simulink model "sim_DOF"  (R2020a)
settings: Solver=ode4  StartTime=0  StopTime=t_end  FixedStep=Step_Time  RelTol=1e-3
values from neighbouring files (symbols this model uses):
  A = [ 0 1 ... (first row only)    [hils2.m]    (also in miniHILS_data.m = [ 0 0 1 0; model_DOF.m = 0.003)
  c1 = 140    [model_DOF.m]    (also in model_nonfeedback.m = 7)
  c2 = 1000    [hils2.m]    (also in miniHILS_data.m = 7; model_DOF.m = 37; model_nonfeedback.m = 13)
  Hz = 2*2*pi    (= 12.5663706144)    [model_DOF.m]
  k1 = 180000    [hils2.m]    (also in miniHILS_data.m = 2200; model_DOF.m = 2200; model_nonfeedback.m = 2200)
  k2 = 30000    [hils2.m]    (also in miniHILS_data.m = 405; model_DOF.m = 405; model_nonfeedback.m = 405)
  m1 = 30.0    (= 30)    [hils2.m]    (also in miniHILS_data.m = 1.5; model_DOF.m = 1.5; model_nonfeedback.m = 1.5)
  m2 = 300.0    (= 300)    [hils2.m]    (also in miniHILS_data.m = 6.4; model_DOF.m = 6.4; model_nonfeedback.m = 6.4)
  T_diff = 1/(2*pi*cutoff)    (= 0.00795774715459)    [miniHILS_data.m]    (also in model_DOF.m = 0.00198943678865)
settings Model: Creator=Peanatsu  LastModifiedBy=Natsu Nakagawa

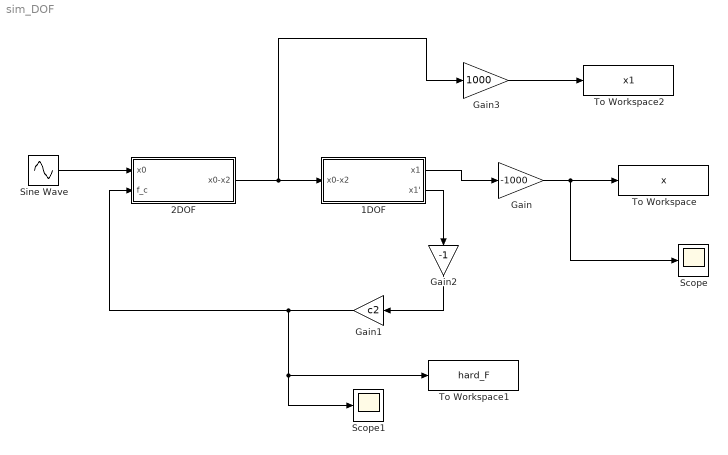
== system sim_DOF ==
  1DOF : Subsystem
  2DOF : Subsystem
  Gain : Gain  Gain=-1000
  Gain1 : Gain  Gain=c2
  Gain2 : Gain  Gain=-1
  Gain3 : Gain  Gain=1000
  Scope : Scope
  Scope1 : Scope
  Sine Wave : Sin  Amplitude=A  Frequency=Hz  SampleTime=0
  To Workspace : ToWorkspace  VariableName=x  SaveFormat=Timeseries  SampleTime=-1
  To Workspace1 : ToWorkspace  VariableName=hard_F  SaveFormat=Timeseries  SampleTime=-1
  To Workspace2 : ToWorkspace  VariableName=x1  SaveFormat=Timeseries  SampleTime=-1
  wires:
  Gain/1 -> Scope/1, To Workspace/1
  1DOF/1(x1) -> Gain/1
  Sine Wave/1 -> 2DOF/1(x0)
  1DOF/2(x1') -> Gain2/1
  Gain1/1 -> To Workspace1/1, Scope1/1, 2DOF/2(f_c)
  Gain2/1 -> Gain1/1
  Gain3/1 -> To Workspace2/1
  2DOF/1(x0-x2) -> Gain3/1, 1DOF/1(x0-x2)

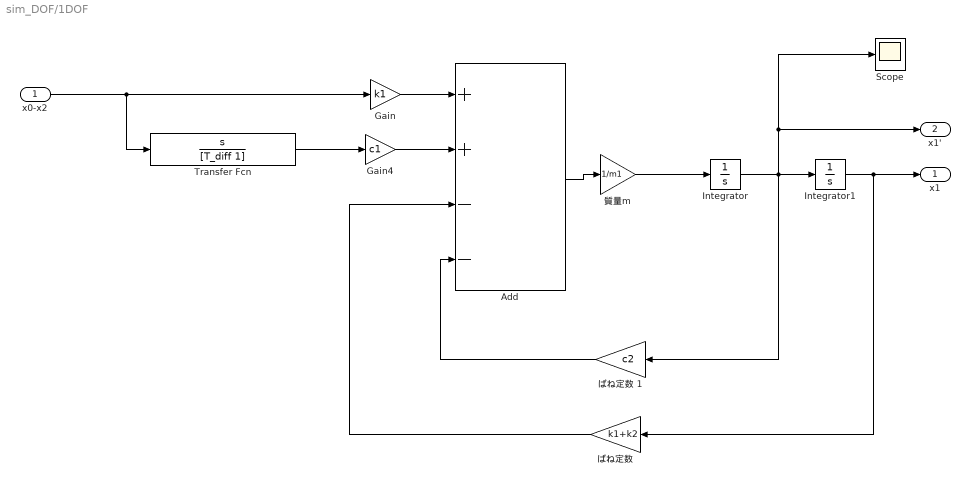
== system sim_DOF/1DOF ==
  x0-x2 : Inport
  Add : Sum  Inputs=++--
  Gain : Gain  Gain=k1
  Gain4 : Gain  Gain=c1
  Integrator : Integrator
  Integrator1 : Integrator
  Scope : Scope
  Transfer Fcn : TransferFcn  Numerator=[1 0]  Denominator=[T_diff 1]
  "ばね定数 " : Gain  Gain=k1+k2
  ばね定数 1 : Gain  Gain=c2
  質量m : Gain  Gain=1/m1
  x1 : Outport
  x1' : Outport  Port=2
  wires:
  Integrator/1 -> ばね定数 1/1, Scope/1, x1'/1, Integrator1/1
  Add/1 -> 質量m/1
  x0-x2/1 -> Transfer Fcn/1, Gain/1
  質量m/1 -> Integrator/1
  Integrator1/1 -> x1/1, "ばね定数 "/1
  Gain/1 -> Add/1
  "ばね定数 "/1 -> Add/3
  Transfer Fcn/1 -> Gain4/1
  Gain4/1 -> Add/2
  ばね定数 1/1 -> Add/4

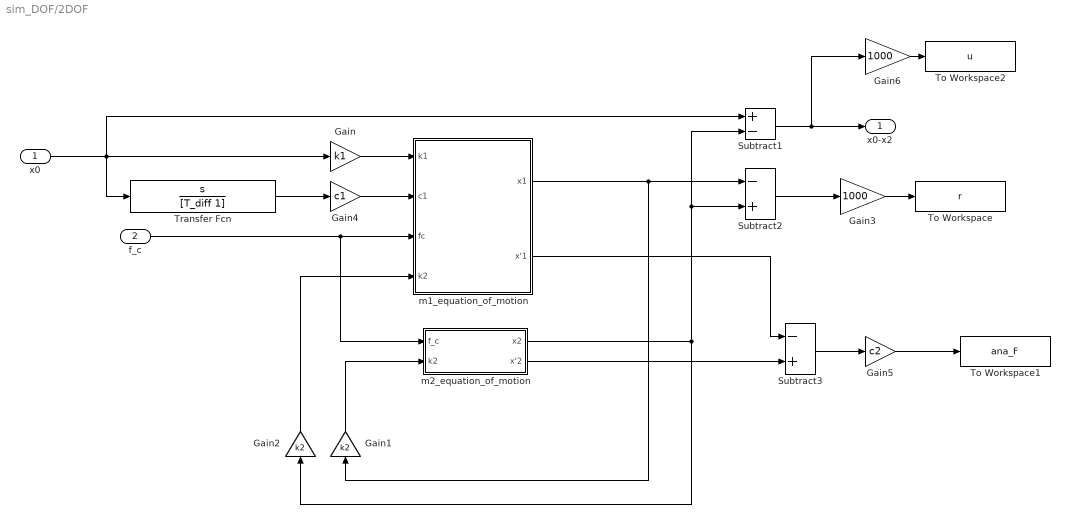
== system sim_DOF/2DOF ==
  x0 : Inport
  f_c : Inport  Port=2
  Gain : Gain  Gain=k1
  Gain1 : Gain  Gain=k2
  Gain2 : Gain  Gain=k2
  Gain3 : Gain  Gain=1000
  Gain4 : Gain  Gain=c1
  Gain5 : Gain  Gain=c2
  Gain6 : Gain  Gain=1000
  Subtract1 : Sum  Inputs=+-
  Subtract2 : Sum  Inputs=-+
  Subtract3 : Sum  Inputs=-+
  To Workspace : ToWorkspace  VariableName=r  SaveFormat=Timeseries  SampleTime=-1
  To Workspace1 : ToWorkspace  VariableName=ana_F  SaveFormat=Timeseries  SampleTime=-1
  To Workspace2 : ToWorkspace  VariableName=u  SaveFormat=Timeseries  SampleTime=-1
  Transfer Fcn : TransferFcn  Numerator=[1 0]  Denominator=[T_diff 1]
  m1_equation_of_motion : Subsystem
  m2_equation_of_motion : Subsystem
  x0-x2 : Outport
  wires:
  x0/1 -> Gain/1, Transfer Fcn/1, Subtract1/1
  Gain/1 -> m1_equation_of_motion/1(k1)
  m1_equation_of_motion/1(x1) -> Gain1/1, Subtract2/1
  Gain1/1 -> m2_equation_of_motion/2("k2 ")
  Subtract2/1 -> Gain3/1
  Gain3/1 -> To Workspace/1
  m2_equation_of_motion/1(x2) -> Gain2/1, Subtract1/2, Subtract2/2
  Gain2/1 -> m1_equation_of_motion/4(k2)
  f_c/1 -> m2_equation_of_motion/1(f_c), m1_equation_of_motion/3(fc)
  Gain4/1 -> m1_equation_of_motion/2(c1)
  Transfer Fcn/1 -> Gain4/1
  Gain5/1 -> To Workspace1/1
  Subtract1/1 -> Gain6/1, x0-x2/1
  Gain6/1 -> To Workspace2/1
  m2_equation_of_motion/2(x'2) -> Subtract3/2
  m1_equation_of_motion/2(x'1) -> Subtract3/1
  Subtract3/1 -> Gain5/1

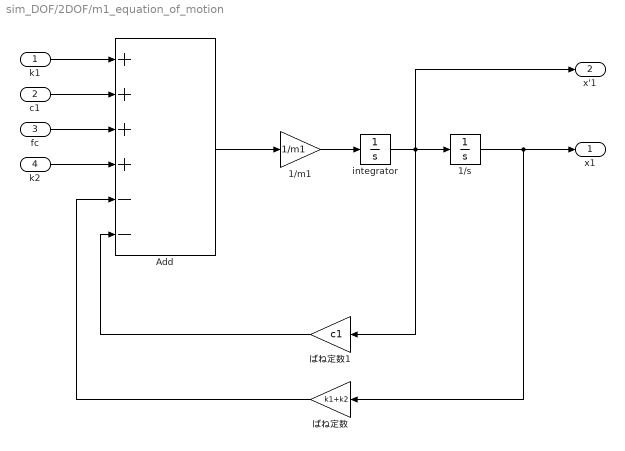
== system sim_DOF/2DOF/m1_equation_of_motion ==
  k1 : Inport
  c1 : Inport  Port=2
  fc : Inport  Port=3
  k2 : Inport  Port=4
  1/m1 : Gain  Gain=1/m1
  1/s : Integrator
  Add : Sum  Inputs=++++--
  integrator : Integrator
  ばね定数 : Gain  Gain=k1+k2
  ばね定数1 : Gain  Gain=c1
  x1 : Outport
  x'1 : Outport  Port=2
  wires:
  k1/1 -> Add/1
  Add/1 -> 1/m1/1
  integrator/1 -> x'1/1, 1/s/1, ばね定数1/1
  1/s/1 -> x1/1, ばね定数/1
  1/m1/1 -> integrator/1
  ばね定数1/1 -> Add/6
  ばね定数/1 -> Add/5
  k2/1 -> Add/4
  c1/1 -> Add/2
  fc/1 -> Add/3

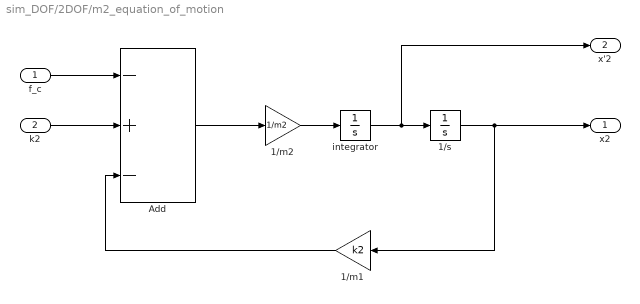
== system sim_DOF/2DOF/m2_equation_of_motion ==
  f_c : Inport
  "k2 " : Inport  Port=2
  1/m1 : Gain  Gain=k2
  1/m2 : Gain  Gain=1/m2
  1/s : Integrator
  Add : Sum  Inputs=-+-
  integrator : Integrator
  x2 : Outport
  x'2 : Outport  Port=2
  wires:
  f_c/1 -> Add/1
  "k2 "/1 -> Add/2
  Add/1 -> 1/m2/1
  integrator/1 -> x'2/1, 1/s/1
  1/s/1 -> 1/m1/1, x2/1
  1/m2/1 -> integrator/1
  1/m1/1 -> Add/3
